simulink model "Test_SG_circuit_exc_turb"  (R2020b)
settings: Solver=ode1  StartTime=0.0  StopTime=15  FixedStep=10e-6  RelTol=1e-3
values from neighbouring files (symbols this model uses):
  L1d_pu = Lb/Lbase    [SG_param.m]    (also in SG_param_tool.m; SG_param_tool_POD.m = (Xd_subtr-Xl)*(Lmd_pu*Lfd_pu)/(Lmd_pu*Lfd_pu-(Lfd_pu+Lmd_pu))
  L1q_pu = La/Lbase    [SG_param.m]    (also in SG_param_tool.m; SG_param_tool_POD.m = (Lmq_pu*(Xq_tr-Xl))/(Lmq_pu-Xq_tr+Xl))
  L2q_pu = Lb/Lbase    [SG_param.m]    (also in SG_param_tool.m; SG_param_tool_POD.m = (Xq_subtr-Xl)*(Lmq_pu*L1q_pu)/(Lmq_pu*L1q_pu-(L1q_pu+Lmq_pu))
  Lfd_pu = La/Lbase    [SG_param.m]    (also in SG_param_tool.m; SG_param_tool_POD.m = (Lmd_pu*(Xd_tr-Xl))/(Lmd_pu-Xd_tr+Xl))
  Ll_pu = Xl    (= 0.2)    [SG_param.m]    (also in SG_param_tool.m; SG_param_tool_POD.m = Xl)
  Lmd_pu = Xd - Xl    (= 1.6)    [SG_param.m]    (also in SG_param_tool.m; SG_param_tool_POD.m = Xd - Xl)
  Lmq_pu = Xq - Xl    (= 1.5)    [SG_param.m]    (also in SG_param_tool.m; SG_param_tool_POD.m = Xq - Xl)
  Pm = Psg0+(Iq.^2+Id.^2)*Rs_pu    [Init_values_Simulink.m]    (also in Init_values_Simulink_trafo.m)
  R1d_pu = rb/Zb    [SG_param.m]    (also in SG_param_tool.m; SG_param_tool_POD.m = 1/(Tdo_subtr*wb)*(L1d_pu+Lmd_pu*Lfd_pu/(Lmd_pu+Lfd_pu)))
  R1q_pu = ra/Zb    [SG_param.m]    (also in SG_param_tool.m; SG_param_tool_POD.m = (Lmq_pu+L1q_pu)/(Tqo_tr*wb))
  R2q_pu = rb/Zb    [SG_param.m]    (also in SG_param_tool.m; SG_param_tool_POD.m = 1/(Tqo_subtr*wb)*(L2q_pu+Lmq_pu*L1q_pu/(Lmq_pu+L1q_pu)))
  Rf_pu = ra/Zb    [SG_param.m]    (also in SG_param_tool.m; SG_param_tool_POD.m = (Lmd_pu+Lfd_pu)/(Tdo_tr*wb))
  Rs_pu = 0.0025    [SG_param.m]    (also in SG_param_tool.m; SG_param_tool_POD.m)
  Rsnb = 300    [SG_param.m]    (also in SG_param_tool.m; SG_param_tool_POD.m; SS_model_grid.m = Vn^2/(data.SG(ii,2)*1e6*0.01)*Ssnb(ii))
  Vb = 22e3    (= 22000)    [SG_param.m]    (also in sg_slack_POD.m = Vb_kV*1e3)
  Vf = Efd    [Init_values_Simulink.m]    (also in Init_values_Simulink_trafo.m)
  Vref = Efd/Exc.KA+V    [Init_values_Simulink.m]    (also in Init_values_Simulink_trafo.m = Vf/Exc.KA+V; Initial_values_for_linear_model.m = Efd/Exc.KA+abs(Vin))
  wn = 2*pi*fn    (= 314.159265359)    [SG_param.m]
undefined symbols (not defined in the file or in its folder): Exc, Lg, Rg, tstep
libraries: powerlib x41, simulink_extras x9, powerlib_meascontrol x2
(part 1 of 2)
settings Model: Creator=Usuario  LastModifiedBy=Collados

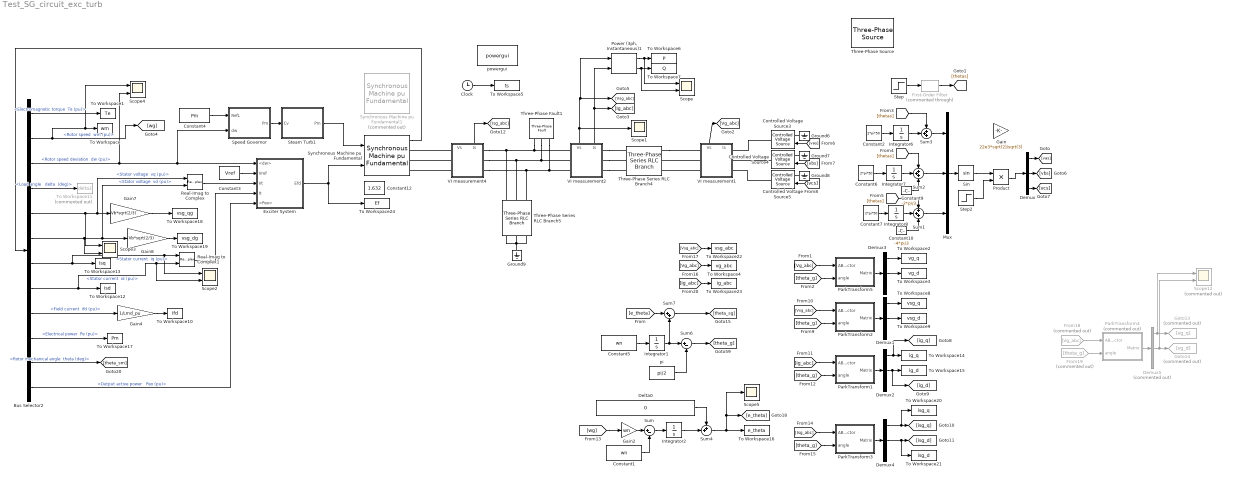
== system Test_SG_circuit_exc_turb ==
  Bus Selector2 : BusSelector  OutputSignals="Mechanical.Electromagnetic torque  Te (pu),Mechanical.Rotor speed  wm (pu),Mechanical.Rotor speed deviation  dw (pu),Load angle   delta  (deg),dq0 components.Stator voltage  vq (pu),dq0 components.Stator voltage  vd (pu),dq0 components.Stator current  iq (pu),dq0 components.Stator current  id (pu),dq0 components.Field current  ifd (pu),Mechanical.Electrical power  Pe (pu),Mechanical.Rotor mechanical angle  theta (deg),Output active power   Peo (pu)"
  Clock : Clock
  Constant1 : Constant  Value=wn
  Constant10 : Constant  Value=-4*pi/3
  Constant12 : Constant  Value=1.632
  Constant2 : Constant  Value=2*pi*50
  Constant3 : Constant  Value=Vref
  Constant4 : Constant  Value=Pm
  Constant5 : Constant  Value=wn
  Constant6 : Constant  Value=2*pi*50
  Constant7 : Constant  Value=2*pi*50
  Constant9 : Constant  Value=-2*pi/3
  Controlled Voltage Source3 : powerlib/Electrical Sources/Controlled Voltage Source  Initialize=on  Source_Type=AC  Amplitude=0  Phase=0  Frequency=0  Measurements=None
  Controlled Voltage Source4 : powerlib/Electrical Sources/Controlled Voltage Source  Initialize=on  Source_Type=AC  Amplitude=0  Phase=0  Frequency=0  Measurements=None
  Controlled Voltage Source5 : powerlib/Electrical Sources/Controlled Voltage Source  Initialize=on  Source_Type=AC  Amplitude=0  Phase=0  Frequency=0  Measurements=None
  Delta0 : Constant  Value=0
  Demux{,1..4} (5 alike) : Demux  Outputs=3
  Demux5 : Demux  Commented=on  Outputs=3
  Exciter System : Subsystem
  First-Order Filter : powerlib_meascontrol/Filters/First-Order Filter  Commented=through  FilterType=Lowpass  Tc=41.4e-3  Ts=0  Initialize=off  Vac_Init=[0, 0, 60]  Vdc_Init=0  PlotResponse=off  FreqRange="[0,  200,  1]"
  From18 : From  Commented=on  GotoTag=Vg_abc
  From19 : From  Commented=on  GotoTag=theta_g
  Gain : Gain  Gain=22e3*sqrt(2)/sqrt(3)
  Gain2 : Gain  Gain=wn
  Gain4 : Gain  Gain=1/Lmd_pu
  Gain7 : Gain  Gain=Vb*sqrt(2/3)
  Gain8 : Gain  Gain=Vb*sqrt(2/3)
  Goto13 : Goto  Commented=on  GotoTag=vg_q
  Goto14 : Goto  Commented=on  GotoTag=vg_d
  Ground{6..9} (4 alike) : powerlib/Elements/Ground  LConnTagsString=a
  Integrator{1..2,6..8} (5 alike) : Integrator
  Mux : Mux  Inputs=3
  ParkTransform1 : Subsystem  mask(Gerard){}
      mask help:
      | This block applies the park transfomation from a desired vector.
      | The input Xabc refers to the vector in the ABC frame, and the second input is the angle used in the transformation.
      | The output is the vector in the qd0 frame.
      mask Display:
      | port_label('output',1,'Xqd0')
      | port_label('input',1,'Xabc')
      | port_label('input',2,'angle')
  ParkTransform2 : Subsystem  mask(Gerard){}
      mask help:
      | This block applies the park transfomation from a desired vector.
      | The input Xabc refers to the vector in the ABC frame, and the second input is the angle used in the transformation.
      | The output is the vector in the qd0 frame.
      mask Display:
      | port_label('output',1,'Xqd0')
      | port_label('input',1,'Xabc')
      | port_label('input',2,'angle')
  ParkTransform3 : Subsystem  mask(Gerard){}
      mask help:
      | This block applies the park transfomation from a desired vector.
      | The input Xabc refers to the vector in the ABC frame, and the second input is the angle used in the transformation.
      | The output is the vector in the qd0 frame.
      mask Display:
      | port_label('output',1,'Xqd0')
      | port_label('input',1,'Xabc')
      | port_label('input',2,'angle')
  ParkTransform4 : Subsystem  Commented=on  mask(Gerard){}
      mask help:
      | This block applies the park transfomation from a desired vector.
      | The input Xabc refers to the vector in the ABC frame, and the second input is the angle used in the transformation.
      | The output is the vector in the qd0 frame.
      mask Display:
      | port_label('output',1,'Xqd0')
      | port_label('input',1,'Xabc')
      | port_label('input',2,'angle')
  ParkTransform5 : Subsystem  mask(Gerard){}
      mask help:
      | This block applies the park transfomation from a desired vector.
      | The input Xabc refers to the vector in the ABC frame, and the second input is the angle used in the transformation.
      | The output is the vector in the qd0 frame.
      mask Display:
      | port_label('output',1,'Xqd0')
      | port_label('input',1,'Xabc')
      | port_label('input',2,'angle')
  "Power (3ph, Instantaneous)1" : powerlib_meascontrol/Measurements/Power (3ph, Instantaneous)
  Product : Product
  Real-Imag to Complex : RealImagToComplex
  Real-Imag to Complex1 : RealImagToComplex
  Scope{,2..4} (4 alike) : Scope  NumInputPorts=2
  Scope1 : Scope
  Scope12 : Scope  Commented=on  NumInputPorts=2
  Scope5 : Scope
  Sin : Trigonometry
  Speed Governor : Subsystem  mask{R=0.05, T1=0.5, T2=3, T3=10, Dt=0, Vmin=0, Vmax=10, P0=Pm}
      mask prompts: R "Controller droop (R)"; T1 "Governor time constant (T1)(sec)"; T2 "Turbine derivative time constant (T2)(sec)"; T3 "Turbine delay time constant (T3)(sec)"; Dt "Frictional losses factor (Dt)"; Vmin "Minimum gate limit (Vmin)(p.u)"; Vmax "Maximum gate limit (Vmax)(p.u)"; P0 "Initial power (p.u)"
      mask Display:
      | disp('TGOV')
      | 
      | port_label('input',1,'Pref')
      | port_label('input',2,'dw')
      | 
      | port_label('output',1,'Cv')
  Steam Turb1 : Subsystem  mask{K1=0.22, K3=0, K5=0.14, K7=0.14, K2=0, K4=0.22, K6=0.14, K8=0.14, T4=0.25, T5=7.5, T6=7.5, T7=0.4, P0=Pm}
      mask prompts: K1 "K1 fraction (HP Turbine)(pu)"; K3 "K3 fraction (HP Turbine)(pu)"; K5 "K5 fraction (HP Turbine)(pu)"; K7 "K7 fraction (HP Turbine)(pu)"; K2 "K2 fraction (LP Turbine)(pu)"; K4 "K4 fraction (LP Turbine)(pu)"; K6 "K6 fraction (LP Turbine)(pu)"; K8 "K8 fraction (LP Turbine)(pu)"; T4 "Steam chest time constant (T4)(sec)"; T5 "Reheater time constant (T5)(sec)"; T6 "Reheater/cross-over time constant (T6)(sec)"; T7 "Cross-over time constant (T7)(sec)"; P0 "Initial power (p.u)"
      mask Display:
      | disp('TTurb')
      | 
      | port_label('input',1,'Cv')
      | 
      | port_label('output',1,'Pm')
  Step : Step  Time=tstep+100  After=10*pi/180  SampleTime=0
  Step2 : Step  Time=tstep  Before=22e3*sqrt(2)/sqrt(3)  After=22e3*sqrt(2)/sqrt(3)*1.005  SampleTime=0
  Sum : Sum  Inputs=|+-
  Sum1 : Sum  Inputs=+++
  Sum2 : Sum  Inputs=+++
  Sum3 : Sum  Inputs=+++
  Sum4 : Sum  Inputs=++|
  Sum6 : Sum  Inputs=|+-
  Sum7 : Sum  Inputs=|++
  Synchronous Machine pu Fundamental : powerlib/Machines/Synchronous Machine pu Fundamental  PresetModel=No  MechanicalLoad=Mechanical power Pm  ShowDetailedParameters=on  RotorType=Round  Units=per unit fundamental parameters  MeasurementBus=off  NominalParameters="[100e6  22e3   50]"  Stator="[Rs_pu  Ll_pu  Lmd_pu  Lmq_pu ]"  Field="[ Rf_pu  Lfd_pu]"  Dampers2=[R1d_pu, L1d_pu, R1q_pu, L1q_pu, R2q_pu, L2q_pu ]  Dampers1="[ 1.17E-02  0.182  1.97E-02  0.384 ]"  Mechanical=[ 5 0 1]  PolePairs=20  InitialConditions=init_values_SG  SetSaturation=off  Saturation=[0.6404,0.7127,0.8441,0.9214,0.9956,1.082,1.19,1.316,1.457;0.7,0.7698,0.8872,0.9466,0.9969,1.046,1.1,1.151,1.201]  LoadFlowParameters=[1,0,0,0,0]  TsPowergui=0  TsBlock=-1  IterativeModel=Trapezoidal non iterative  IterativeDiscreteModel=Trapezoidal non iterative  BusType=PQ  Pref=50e6  Qref=20e6  Qmin=-inf  Qmax=inf  PLF=0  QLF=0
      settings: SourceProductBaseCode=PS
  Synchronous Machine pu Fundamental1 : powerlib/Machines/Synchronous Machine pu Fundamental  Commented=on  PresetModel=No  MechanicalLoad=Mechanical power Pm  ShowDetailedParameters=on  RotorType=Round  Units=per unit fundamental parameters  MeasurementBus=off  NominalParameters="[100e6  22e3   50]"  Stator="[ 0.0025  0.14  1.66  0.91 ]"  Field="[ 0.00043  0.2004]"  Dampers2=[0.0051, 0.0437, 0.00842, 0.106, 8.1942e-3, 9.4199e-2 ]  Dampers1="[ 1.17E-02  0.182  1.97E-02  0.384 ]"  Mechanical=[ 5 0 2]  PolePairs=20  InitialConditions=[0 -78.0791 0.205424 0.205424 0.205424 -13.3134 -133.313 106.687 1.14256]  SetSaturation=off  Saturation=[0.6404,0.7127,0.8441,0.9214,0.9956,1.082,1.19,1.316,1.457;0.7,0.7698,0.8872,0.9466,0.9969,1.046,1.1,1.151,1.201]  LoadFlowParameters=[1,0,0,0,0]  TsPowergui=0  TsBlock=-1  IterativeModel=Trapezoidal non iterative  IterativeDiscreteModel=Trapezoidal non iterative  BusType=PQ  Pref=20e6  Qref=5e6  Qmin=-inf  Qmax=inf  PLF=0  QLF=0
      settings: SourceProductBaseCode=PS
  Three-Phase Series RLC Branch4 : powerlib/Elements/Three-Phase Series RLC Branch  LConnTagsString=A|B|C  RConnTagsString=A|B|C  BranchType=RL  Resistance=Rg  Inductance=Lg  Capacitance=1e-6  Measurements=None
  Three-Phase Series RLC Branch5 : powerlib/Elements/Three-Phase Series RLC Branch  LConnTagsString=A|B|C  RConnTagsString=A|B|C  BranchType=R  Resistance=Rsnb  Inductance=1e-3  Capacitance=1e-6  Measurements=None
  Three-Phase Fault1 : powerlib/Elements/Three-Phase Fault  InitialStates=0  FaultA=on  FaultB=off  FaultC=off  GroundFault=on  SwitchTimes=[101 101.2]  External=off  SwitchStatus=NaN  FaultResistance=50  GroundResistance=0.0000001  SnubberResistance=1e6  SnubberCapacitance=inf  Measurements=None
  Three-Phase Source : powerlib/Electrical Sources/Three-Phase Source  InternalConnection=Yg  VoltagePhases=off  Voltage=(22000)*1  PhaseAngle=0  Voltage_phases=[25e3 25e3 25e3]/sqrt(3)  PhaseAngles_phases=[0 -120 +120]  Frequency=50  NonIdealSource=off  SpecifyImpedance=off  Resistance=0.8929  Inductance=16.58e-3  ShortCircuitLevel=100e6  BaseVoltage=22e3  XRratio=7  BusType=swing  Pref=10e3  Qref=0  Prefabc=[10e3, 10e3, 10e3]  Qrefabc=[0, 0, 0]  Qmin=-inf  Qmax=inf
  To Workspace : ToWorkspace  VariableName=wm  SampleTime=-1
      settings: Decimation=20  Save2DSignal=2-D array (concatenate along first dimension)
  To Workspace1 : ToWorkspace  VariableName=Te  SampleTime=-1
      settings: Decimation=20  Save2DSignal=2-D array (concatenate along first dimension)
  To Workspace10 : ToWorkspace  VariableName=ifd  SampleTime=-1
      settings: Decimation=20  Save2DSignal=2-D array (concatenate along first dimension)
  To Workspace11 : ToWorkspace  Commented=on  VariableName=delta2  SampleTime=-1
      settings: Decimation=20  Save2DSignal=2-D array (concatenate along first dimension)
  To Workspace12 : ToWorkspace  VariableName=isd  SampleTime=-1
      settings: Decimation=20  Save2DSignal=2-D array (concatenate along first dimension)
  To Workspace13 : ToWorkspace  VariableName=isq  SampleTime=-1
      settings: Decimation=20  Save2DSignal=2-D array (concatenate along first dimension)
  To Workspace14 : ToWorkspace  VariableName=ig_q  SampleTime=-1
      settings: Decimation=20  Save2DSignal=2-D array (concatenate along first dimension)
  To Workspace15 : ToWorkspace  VariableName=ig_d  SampleTime=-1
      settings: Decimation=20  Save2DSignal=2-D array (concatenate along first dimension)
  To Workspace16 : ToWorkspace  VariableName=e_theta  SampleTime=-1
      settings: Decimation=20  Save2DSignal=2-D array (concatenate along first dimension)
  To Workspace17 : ToWorkspace  VariableName=Pm  SampleTime=-1
      settings: Decimation=20  Save2DSignal=2-D array (concatenate along first dimension)
  To Workspace18 : ToWorkspace  VariableName=vsg_qg  SampleTime=-1
      settings: Decimation=20  Save2DSignal=2-D array (concatenate along first dimension)
  To Workspace19 : ToWorkspace  VariableName=vsg_dg  SampleTime=-1
      settings: Decimation=20  Save2DSignal=2-D array (concatenate along first dimension)
  To Workspace2 : ToWorkspace  VariableName=vg_q  SampleTime=-1
      settings: Decimation=20  Save2DSignal=2-D array (concatenate along first dimension)
  To Workspace20 : ToWorkspace  VariableName=isg_q  SampleTime=-1
      settings: Decimation=20  Save2DSignal=2-D array (concatenate along first dimension)
  To Workspace21 : ToWorkspace  VariableName=isg_d  SampleTime=-1
      settings: Decimation=20  Save2DSignal=2-D array (concatenate along first dimension)
  To Workspace22 : ToWorkspace  VariableName=vsg_abc  SampleTime=-1
      settings: Decimation=20  Save2DSignal=2-D array (concatenate along first dimension)
  To Workspace23 : ToWorkspace  VariableName=ig_abc  SampleTime=-1
      settings: Decimation=20  Save2DSignal=2-D array (concatenate along first dimension)
  To Workspace24 : ToWorkspace  VariableName=Ef  SampleTime=-1
      settings: Decimation=20  Save2DSignal=2-D array (concatenate along first dimension)
  To Workspace3 : ToWorkspace  VariableName=vg_d  SampleTime=-1
      settings: Decimation=20  Save2DSignal=2-D array (concatenate along first dimension)
  To Workspace4 : ToWorkspace  VariableName=vg_abc  SampleTime=-1
      settings: Decimation=20  Save2DSignal=2-D array (concatenate along first dimension)
  To Workspace5 : ToWorkspace  VariableName=ts  SampleTime=-1
      settings: Decimation=20  Save2DSignal=2-D array (concatenate along first dimension)
  To Workspace6 : ToWorkspace  VariableName=P  SampleTime=-1
      settings: Decimation=20  Save2DSignal=2-D array (concatenate along first dimension)
  To Workspace7 : ToWorkspace  VariableName=Q  SampleTime=-1
      settings: Decimation=20  Save2DSignal=2-D array (concatenate along first dimension)
  To Workspace8 : ToWorkspace  VariableName=vsg_q  SampleTime=-1
      settings: Decimation=20  Save2DSignal=2-D array (concatenate along first dimension)
  To Workspace9 : ToWorkspace  VariableName=vsg_d  SampleTime=-1
      settings: Decimation=20  Save2DSignal=2-D array (concatenate along first dimension)
  VI measurement1 : Subsystem
      settings: PortSchema="{\"entries\":[{\"content\":{\"sides\":[{\"content\":{\"connectorIds\":[\"LConn1\",\"LConn2\",\"LConn3\"]},\"type\":\"ConnectorPlacement.EquallySpacedRectSide\",\"uuid\":\"d0d5b0b8-afec-4f90-9eba-536a06b10059\"},{\"content\":{\"connectorIds\":[\"RConn1\",\"RConn2\",\"RConn3\"],\"side\":\"RIGHT\"},\"type\":\"ConnectorPlacement.EquallySpacedRectSide\",\"uuid\":\"adc1b68d-6172-4507-b54b-9373921355a1\"},{\"content\":{\"connectorIds\":[\"Out1\",\"Out2\"],\"side\":\"TOP\"},\"type\":\"ConnectorPlacement.EquallySpacedRectSide\",\"uuid\":\"8c5adf07-e95b-4907-94c3-1b2a47d47f40\"}]},\"type\":\"ConnectorPlacement.EquallySpacedConnector\",\"uuid\":\"87d0b20f-8f85-4790-a611-3415e642a83a\"}],\"packageUris\":[\"http://schema.mathworks.com/mf0/Connector/R2020b\"],\"version\":\"1.0\"}"
  VI measurement2 : Subsystem
      settings: PortSchema="{\"entries\":[{\"content\":{\"sides\":[{\"content\":{\"connectorIds\":[\"LConn1\",\"LConn2\",\"LConn3\"]},\"type\":\"ConnectorPlacement.EquallySpacedRectSide\",\"uuid\":\"d0d5b0b8-afec-4f90-9eba-536a06b10059\"},{\"content\":{\"connectorIds\":[\"RConn1\",\"RConn2\",\"RConn3\"],\"side\":\"RIGHT\"},\"type\":\"ConnectorPlacement.EquallySpacedRectSide\",\"uuid\":\"adc1b68d-6172-4507-b54b-9373921355a1\"},{\"content\":{\"connectorIds\":[\"Out1\",\"Out2\"],\"side\":\"TOP\"},\"type\":\"ConnectorPlacement.EquallySpacedRectSide\",\"uuid\":\"8c5adf07-e95b-4907-94c3-1b2a47d47f40\"}]},\"type\":\"ConnectorPlacement.EquallySpacedConnector\",\"uuid\":\"87d0b20f-8f85-4790-a611-3415e642a83a\"}],\"packageUris\":[\"http://schema.mathworks.com/mf0/Connector/R2020b\"],\"version\":\"1.0\"}"
  VI measurement4 : Subsystem
      settings: PortSchema="{\"entries\":[{\"content\":{\"sides\":[{\"content\":{\"connectorIds\":[\"LConn1\",\"LConn2\",\"LConn3\"]},\"type\":\"ConnectorPlacement.EquallySpacedRectSide\",\"uuid\":\"d0d5b0b8-afec-4f90-9eba-536a06b10059\"},{\"content\":{\"connectorIds\":[\"RConn1\",\"RConn2\",\"RConn3\"],\"side\":\"RIGHT\"},\"type\":\"ConnectorPlacement.EquallySpacedRectSide\",\"uuid\":\"adc1b68d-6172-4507-b54b-9373921355a1\"},{\"content\":{\"connectorIds\":[\"Out1\",\"Out2\"],\"side\":\"TOP\"},\"type\":\"ConnectorPlacement.EquallySpacedRectSide\",\"uuid\":\"8c5adf07-e95b-4907-94c3-1b2a47d47f40\"}]},\"type\":\"ConnectorPlacement.EquallySpacedConnector\",\"uuid\":\"87d0b20f-8f85-4790-a611-3415e642a83a\"}],\"packageUris\":[\"http://schema.mathworks.com/mf0/Connector/R2020b\"],\"version\":\"1.0\"}"
  pi : Constant  Value=pi/2
  powergui : powerlib/powergui  Priority=1  SimulationMode=Discrete  SampleTime=10e-6  frequency=60  Iterations=50  frequencyindice=0  Pbase=100e6  ErrMax=0.0001  UnitsV=kV  UnitsW=MW  buscounter=0  FunctionMessages=off  echomessages=off  EnableUseOfTLC=off  CurrentSourceSwitches=off  DisableSnubberDevices=off  DisableRonSwitches=off  DisableVfSwitches=off  DisplayEquations=off  AutomaticDiscreteSolvers=off  SolverType=Tustin/Backward Euler (TBE)  Interpol=off  ExternalGateDelay=off  methode=off  Ts=100  x0status=blocks  SPID=on  SwTol=0  HookPort=off  NonlinearTolerance=1e-4  nMaxIteration=100  ContinueOnMaxIteration=off  RestoreLinks=warning  ResistiveCurrentMeasurement=off  Frange=[0:2:500]  Ylog=off  Xlog=on  ShowGrid=off  save=off  variable=ZData  structure=0  ZoomFFT=off  StartTime=0.0  cycles=1  DisplayStyle=1  fundamental=60  FreqAxis=off  MaxFrequency=1000  frequencyindicesteady=1  RmsSteady=1  display=off
  wires:
  Constant6/1 -> Integrator7/1
  Demux/3 -> [vcs]
  Demux/1 -> [vas]
  Constant7/1 -> Integrator8/1
  Demux/2 -> [vbs]
  Sum2/1 -> Mux/2
  Sin/1 -> Product/1
  Product/1 -> Demux/1
  Sum1/1 -> Mux/3
  Mux/1 -> Sin/1
  Constant2/1 -> Integrator6/1
  Constant9/1 -> Sum2/3
  Integrator7/1 -> Sum2/2
  Integrator6/1 -> Sum3/2
  [thetas] -> Sum3/1
  [thetas] -> Sum2/1
  Integrator8/1 -> Sum1/2
  Constant10/1 -> Sum1/3
  [thetas] -> Sum1/1
  Sum3/1 -> Mux/1
  Step/1 -> First-Order Filter/1
  First-Order Filter/1 -> [thetas]
  Clock/1 -> To Workspace5/1
  Steam Turb1/1(Pm) -> Synchronous Machine pu Fundamental/1
  [vas] -> Controlled Voltage Source3/1
  [vcs] -> Controlled Voltage Source5/1
  [vbs] -> Controlled Voltage Source4/1
  VI measurement2/2(Is) -> "Power (3ph, Instantaneous)1"/2, [Ig_abc]
  Constant5/1 -> Integrator1/1
  ParkTransform2/1(Matrix) -> Demux1/1
  Integrator1/1 -> Sum6/1, Sum7/2
  [theta_g] -> ParkTransform2/2(angle)
  [Vsg_abc] -> ParkTransform2/1(ABC vector)
  Demux1/2 -> To Workspace9/1
  Demux1/1 -> To Workspace8/1
  Demux2/1 -> [ig_q], To Workspace14/1
  Demux2/2 -> [ig_d], To Workspace15/1
  [Ig_abc] -> ParkTransform1/1(ABC vector)
  [theta_g] -> ParkTransform1/2(angle)
  ParkTransform1/1(Matrix) -> Demux2/1
  VI measurement2/1(Vs) -> Scope1/1, "Power (3ph, Instantaneous)1"/1, [Vsg_abc]
  "Power (3ph, Instantaneous)1"/1 -> Scope/1, To Workspace6/1
  "Power (3ph, Instantaneous)1"/2 -> Scope/2, To Workspace7/1
  [wg] -> Gain2/1
  Sum/1 -> Integrator2/1
  Integrator2/1 -> Sum4/2
  Gain2/1 -> Sum/1
  Sum4/1 -> Scope5/1, [e_theta], To Workspace16/1
  ParkTransform3/1(Matrix) -> Demux4/1
  [theta_g] -> ParkTransform3/2(angle)
  [Isg_abc] -> ParkTransform3/1(ABC vector)
  Demux4/2 -> To Workspace21/1, [isg_d]
  Demux4/1 -> To Workspace20/1, [isg_q]
  VI measurement4/2(Is) -> [Isg_abc]
  From18/1 -> ParkTransform4/1(ABC vector)
  From19/1 -> ParkTransform4/2(angle)
  ParkTransform4/1(Matrix) -> Demux5/1
  Demux5/1 -> Scope12/1, Goto13/1
  Demux5/2 -> Scope12/2, Goto14/1
  pi/1 -> Sum6/2
  Sum6/1 -> [theta_g]
  Sum7/1 -> [theta_sg]
  Step2/1 -> Product/2
  Delta0/1 -> Sum4/1
  Constant1/1 -> Sum/2
  [e_theta] -> Sum7/1
  VI measurement1/1(Vs) -> [Vg_abc]
  Demux3/1 -> To Workspace2/1
  Demux3/2 -> To Workspace3/1
  [Vg_abc] -> ParkTransform5/1(ABC vector)
  [theta_g] -> ParkTransform5/2(angle)
  ParkTransform5/1(Matrix) -> Demux3/1
  [Vg_abc] -> To Workspace4/1
  [Vsg_abc] -> To Workspace22/1
  [Ig_abc] -> To Workspace23/1
  Bus Selector2/10 -> To Workspace17/1  "<Electrical power  Pe (pu)>"
  Real-Imag to Complex1/1 -> Exciter System/4(It)
  Gain7/1 -> To Workspace18/1
  Bus Selector2/9 -> Gain4/1  "<Field current  ifd (pu)>"
  Constant3/1 -> Exciter System/2(Vref)
  Bus Selector2/6 -> Scope3/2, Real-Imag to Complex/2, Gain8/1  "<Stator voltage  vd (pu)>"
  Bus Selector2/1 -> To Workspace1/1  "<Electromagnetic torque  Te (pu)>"
  Bus Selector2/5 -> Scope3/1, Real-Imag to Complex/1, Gain7/1  "<Stator voltage  vq (pu)>"
  Bus Selector2/7 -> Scope2/1, Real-Imag to Complex1/1, To Workspace13/1  "<Stator current  iq (pu)>"
  Bus Selector2/4 -> To Workspace11/1  "<Load angle   delta  (deg)>"
  Synchronous Machine pu Fundamental/1 -> Bus Selector2/1
  Bus Selector2/2 -> Scope4/1, To Workspace/1, [wg]  "<Rotor speed  wm (pu)>"
  Bus Selector2/11 -> [theta_sm]  "<Rotor mechanical angle  theta (deg)>"
  Real-Imag to Complex/1 -> Exciter System/3(Vt)
  Gain8/1 -> To Workspace19/1
  Gain4/1 -> To Workspace10/1
  Bus Selector2/8 -> Scope2/2, Real-Imag to Complex1/2, To Workspace12/1  "<Stator current  id (pu)>"
  Bus Selector2/12 -> Exciter System/5(<Peo>)  "<Output active power   Peo (pu)>"
  Exciter System/1(Efd) -> Synchronous Machine pu Fundamental/2, To Workspace24/1
  Constant4/1 -> Speed Governor/1(RefL)
  Bus Selector2/3 -> Scope4/2, Speed Governor/2(dw), Exciter System/1(<dw>)  "<Rotor speed deviation  dw (pu)>"
  Speed Governor/1(Pm) -> Steam Turb1/1(Cv)
  connections:
  Three-Phase Fault1/LConn1 -- VI measurement2/LConn1 -- Three-Phase Series RLC Branch5/LConn1 -- VI measurement4/RConn1
  Three-Phase Series RLC Branch5/RConn1 -- Ground9/LConn1 -- Three-Phase Series RLC Branch5/RConn2 -- Three-Phase Series RLC Branch5/RConn3
  Ground6/LConn1 -- Controlled Voltage Source3/LConn1
  VI measurement2/RConn2 -- Three-Phase Series RLC Branch4/LConn2
  Ground7/LConn1 -- Controlled Voltage Source4/LConn1
  Ground8/LConn1 -- Controlled Voltage Source5/LConn1
  VI measurement2/RConn3 -- Three-Phase Series RLC Branch4/LConn3
  VI measurement2/RConn1 -- Three-Phase Series RLC Branch4/LConn1
  VI measurement4/LConn1 -- Synchronous Machine pu Fundamental/RConn1
  VI measurement4/LConn2 -- Synchronous Machine pu Fundamental/RConn2
  VI measurement4/LConn3 -- Synchronous Machine pu Fundamental/RConn3
  VI measurement4/RConn2 -- VI measurement2/LConn2 -- Three-Phase Fault1/LConn2 -- Three-Phase Series RLC Branch5/LConn2
  VI measurement4/RConn3 -- VI measurement2/LConn3 -- Three-Phase Fault1/LConn3 -- Three-Phase Series RLC Branch5/LConn3
  Three-Phase Series RLC Branch4/RConn1 -- VI measurement1/LConn1
  Controlled Voltage Source3/RConn1 -- VI measurement1/RConn1
  Controlled Voltage Source4/RConn1 -- VI measurement1/RConn2
  Controlled Voltage Source5/RConn1 -- VI measurement1/RConn3
  VI measurement1/LConn2 -- Three-Phase Series RLC Branch4/RConn2
  VI measurement1/LConn3 -- Three-Phase Series RLC Branch4/RConn3

== system Test_SG_circuit_exc_turb/Exciter System ==
  <dw> : Inport
  Vref : Inport  Port=2
  Vt : Inport  Port=3
  It : Inport  Port=4
  <Peo> : Inport  Port=5
  PSS1 : Subsystem  mask{Ks1=20, Ks2=0.1564, Ks3=1, Tw1=2, Tw2=2, Tw3=2, Tw4=0, T1=0.25, T2=0.2, T3=0.15, T4=0.1, T6=0, T7=2, T8=0.5, T9=0.1, Vstmin=-0.10, Vstmax=0.10, N=1, M=1, IC1=1, IC2=3}
      mask prompts: Ks1 "PSS gain (Ks1)"; Ks2 "2nd signal transducer factor(Ks2)"; Ks3 "washouts coupling factor (Ks3)"; Tw1 "1st washout 1th time constant (Tw1)(sec)"; Tw2 "1st washout 2nd time constant (Tw2)(sec)"; Tw3 "2nd washout 1st time constant (Tw3)(sec)"; Tw4 "2nd washout 2nd time constant (Tw4)(sec)"; T1 "1st lead-lag derivative time constant (T1)(sec)"; T2 "1st lead-lag delay time constant(T2)(sec)"; T3 "2nd lead-lag derivative time constant(T3)(sec)"; T4 "2nd lead-lag delay time constant(T4)(sec)"; T6 "1st signal transducer time constant(T6)(sec)"; T7 "2nd signal transducer time constant(T7)(sec)"; T8 "ramp tracking filter deriv. time constant(T8)(sec)"; T9 "ramp tracking filter delay time constant(T9)(sec)"; Vstmin "controller minimum output(Vstmin)"; Vstmax "controller maximum output(Vstmax)"; N "ramp tracking filter (N)"; M "ramp tracking filter (M)"; IC1 "1st input selector (IC1)"; IC2 "2nd input selector (IC2)"
      mask Display:
      | disp('PSS2A')
      | 
      | port_label('input',1,'dw')
      | port_label('input',2,'Pg')
      | %port_label('input',3,'Vs')
      | 
      | port_label('output',1,'Vs')
  PSS1 backup : Subsystem  Commented=on  mask{Ks1=10, Ks2=0.1564, Ks3=1, Tw1=2, Tw2=2, Tw3=2, Tw4=0, T1=0.25, T2=0.03, T3=0.15, T4=0.015, T6=0, T7=2, T8=0.5, T9=0.1, Vstmin=-0.1, Vstmax=0.1, N=0, M=0, IC1=1, IC2=3}
      mask prompts: Ks1 "PSS gain (Ks1)"; Ks2 "2nd signal transducer factor(Ks2)"; Ks3 "washouts coupling factor (Ks3)"; Tw1 "1st washout 1th time constant (Tw1)(sec)"; Tw2 "1st washout 2nd time constant (Tw2)(sec)"; Tw3 "2nd washout 1st time constant (Tw3)(sec)"; Tw4 "2nd washout 2nd time constant (Tw4)(sec)"; T1 "1st lead-lag derivative time constant (T1)(sec)"; T2 "1st lead-lag delay time constant(T2)(sec)"; T3 "2nd lead-lag derivative time constant(T3)(sec)"; T4 "2nd lead-lag delay time constant(T4)(sec)"; T6 "1st signal transducer time constant(T6)(sec)"; T7 "2nd signal transducer time constant(T7)(sec)"; T8 "ramp tracking filter deriv. time constant(T8)(sec)"; T9 "ramp tracking filter delay time constant(T9)(sec)"; Vstmin "controller minimum output(Vstmin)"; Vstmax "controller maximum output(Vstmax)"; N "ramp tracking filter (N)"; M "ramp tracking filter (M)"; IC1 "1st input selector (IC1)"; IC2 "2nd input selector (IC2)"
      mask Display:
      | disp('PSS2A')
      | 
      | port_label('input',1,'dw')
      | port_label('input',2,'Pg')
      | %port_label('input',3,'Vs')
      | 
      | port_label('output',1,'Vs')
  SEXS1 : Subsystem  mask{K=Exc.KA, Ta=Exc.TC, Tb=Exc.TB, Te=Exc.TA, Emin=Exc.VRmin, Emax=Exc.VRmax, Vf0=Vf}
      mask prompts: K "Controller gain (K)"; Ta "Filter derivative time constant (Ta)(sec)"; Tb "Filter delay time (Tb)(sec)"; Te "Exciter time constant (Te)(sec)"; Emin "Controller minimum output (Emin)"; Emax "Controller maximum output (Emax)"; Vf0 "Initial value of field voltage"
      mask Display:
      | disp('AVR')
      | 
      | port_label('input',1,'Vref')
      | port_label('input',2,'Vc')
      | port_label('input',3,'Vs')
      | 
      | port_label('output',1,'Efd')
  TR and LC_test : Subsystem  mask{Tr=10e-3, Rc=0, Xc=0}
      mask prompts: Tr "Transducter filter time constant (Tr)(sec)"; Rc "Resistance to compensate (p.u)"; Xc "Reactance to compensate (p.u)"
      mask Display:
      | %disp('Transducer \n \n')
      | %disp('and \n')
      | %disp('Load compensation')
      | text(15,35, 'Transducer')
      | text(30,24, 'and')
      | text(15,14, 'Load comp')
      | 
      | port_label('input',1,'Vt')
      | port_label('input',2,'It')
      | 
      | port_label('output',1,'Vc')
  To Workspace24 : ToWorkspace  VariableName=Vsg_mag  SampleTime=-1
      settings: Decimation=20  Save2DSignal=2-D array (concatenate along first dimension)
  Efd : Outport
  wires:
  SEXS1/1(Efd) -> Efd/1
  It/1 -> TR and LC_test/2(It)
  PSS1/1(Vothsg) -> ?
  <Peo>/1 -> PSS1/2(Pgen)
  <dw>/1 -> PSS1/1(dw)
  Vt/1 -> TR and LC_test/1(Vt)
  Vref/1 -> SEXS1/1(Vref)
  TR and LC_test/1(Vc) -> To Workspace24/1, SEXS1/2(Vc)

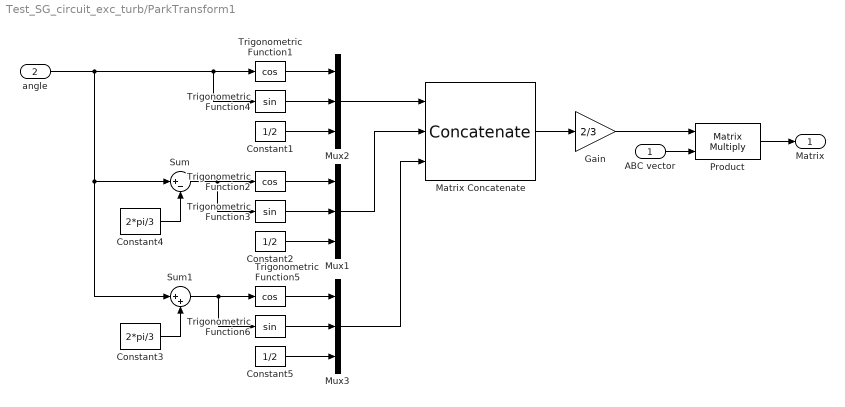
== system Test_SG_circuit_exc_turb/ParkTransform1 ==
  ABC vector : Inport
  angle : Inport  Port=2
  Constant1 : Constant  Value=1/2
  Constant2 : Constant  Value=1/2
  Constant3 : Constant  Value=2*pi/3
  Constant4 : Constant  Value=2*pi/3
  Constant5 : Constant  Value=1/2
  Gain : Gain  Gain=2/3
  Matrix Concatenate : Concatenate  NumInputs=3  Mode=Multidimensional array  ConcatenateDimension=2
  Mux1 : Mux  Inputs=3
  Mux2 : Mux  Inputs=3
  Mux3 : Mux  Inputs=3
  Product : Product  Multiplication=Matrix(*)  RndMeth=Zero
  Sum : Sum  Inputs=|+-
  Sum1 : Sum  Inputs=|++
  Trigonometric Function1 : Trigonometry  Operator=cos
  Trigonometric Function2 : Trigonometry  Operator=cos
  Trigonometric Function3 : Trigonometry
  Trigonometric Function4 : Trigonometry
  Trigonometric Function5 : Trigonometry  Operator=cos
  Trigonometric Function6 : Trigonometry
  Matrix : Outport
  wires:
  Matrix Concatenate/1 -> Gain/1
  ABC vector/1 -> Product/2
  Product/1 -> Matrix/1
  Gain/1 -> Product/1
  Constant4/1 -> Sum/2
  Constant3/1 -> Sum1/2
  angle/1 -> Trigonometric Function4/1, Trigonometric Function1/1, Sum1/1, Sum/1
  Trigonometric Function3/1 -> Mux1/2
  Trigonometric Function2/1 -> Mux1/1
  Constant2/1 -> Mux1/3
  Sum/1 -> Trigonometric Function3/1, Trigonometric Function2/1
  Trigonometric Function4/1 -> Mux2/2
  Trigonometric Function1/1 -> Mux2/1
  Constant1/1 -> Mux2/3
  Trigonometric Function6/1 -> Mux3/2
  Trigonometric Function5/1 -> Mux3/1
  Constant5/1 -> Mux3/3
  Sum1/1 -> Trigonometric Function6/1, Trigonometric Function5/1
  Mux1/1 -> Matrix Concatenate/2
  Mux2/1 -> Matrix Concatenate/1
  Mux3/1 -> Matrix Concatenate/3

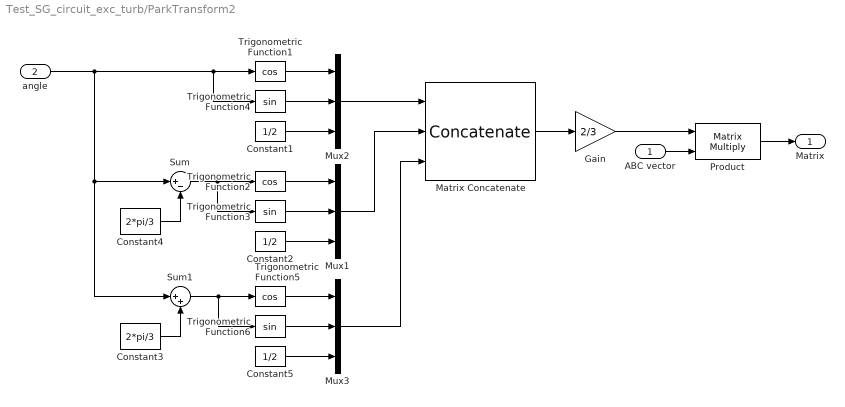
== system Test_SG_circuit_exc_turb/ParkTransform2 ==
  ABC vector : Inport
  angle : Inport  Port=2
  Constant1 : Constant  Value=1/2
  Constant2 : Constant  Value=1/2
  Constant3 : Constant  Value=2*pi/3
  Constant4 : Constant  Value=2*pi/3
  Constant5 : Constant  Value=1/2
  Gain : Gain  Gain=2/3
  Matrix Concatenate : Concatenate  NumInputs=3  Mode=Multidimensional array  ConcatenateDimension=2
  Mux1 : Mux  Inputs=3
  Mux2 : Mux  Inputs=3
  Mux3 : Mux  Inputs=3
  Product : Product  Multiplication=Matrix(*)  RndMeth=Zero
  Sum : Sum  Inputs=|+-
  Sum1 : Sum  Inputs=|++
  Trigonometric Function1 : Trigonometry  Operator=cos
  Trigonometric Function2 : Trigonometry  Operator=cos
  Trigonometric Function3 : Trigonometry
  Trigonometric Function4 : Trigonometry
  Trigonometric Function5 : Trigonometry  Operator=cos
  Trigonometric Function6 : Trigonometry
  Matrix : Outport
  wires:
  Mux3/1 -> Matrix Concatenate/3
  Mux2/1 -> Matrix Concatenate/1
  Mux1/1 -> Matrix Concatenate/2
  Sum1/1 -> Trigonometric Function5/1, Trigonometric Function6/1
  Constant5/1 -> Mux3/3
  Trigonometric Function5/1 -> Mux3/1
  Trigonometric Function6/1 -> Mux3/2
  Constant1/1 -> Mux2/3
  Trigonometric Function1/1 -> Mux2/1
  Trigonometric Function4/1 -> Mux2/2
  Sum/1 -> Trigonometric Function2/1, Trigonometric Function3/1
  Constant2/1 -> Mux1/3
  Trigonometric Function2/1 -> Mux1/1
  Trigonometric Function3/1 -> Mux1/2
  angle/1 -> Sum/1, Sum1/1, Trigonometric Function1/1, Trigonometric Function4/1
  Constant3/1 -> Sum1/2
  Constant4/1 -> Sum/2
  Gain/1 -> Product/1
  Product/1 -> Matrix/1
  ABC vector/1 -> Product/2
  Matrix Concatenate/1 -> Gain/1

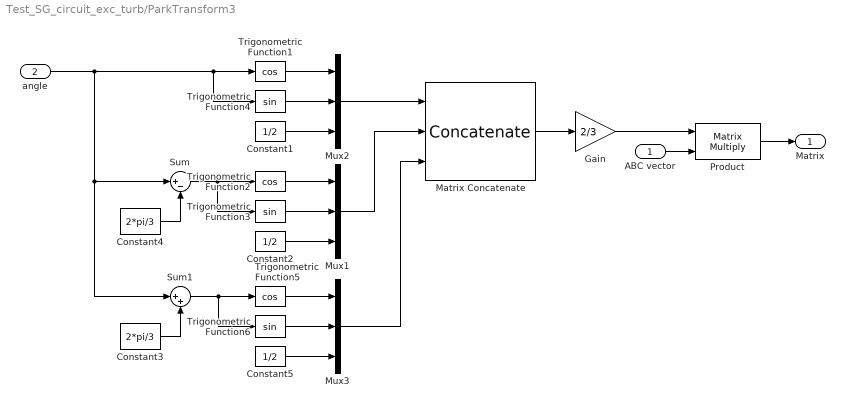
== system Test_SG_circuit_exc_turb/ParkTransform3 ==
  ABC vector : Inport
  angle : Inport  Port=2
  Constant1 : Constant  Value=1/2
  Constant2 : Constant  Value=1/2
  Constant3 : Constant  Value=2*pi/3
  Constant4 : Constant  Value=2*pi/3
  Constant5 : Constant  Value=1/2
  Gain : Gain  Gain=2/3
  Matrix Concatenate : Concatenate  NumInputs=3  Mode=Multidimensional array  ConcatenateDimension=2
  Mux1 : Mux  Inputs=3
  Mux2 : Mux  Inputs=3
  Mux3 : Mux  Inputs=3
  Product : Product  Multiplication=Matrix(*)  RndMeth=Zero
  Sum : Sum  Inputs=|+-
  Sum1 : Sum  Inputs=|++
  Trigonometric Function1 : Trigonometry  Operator=cos
  Trigonometric Function2 : Trigonometry  Operator=cos
  Trigonometric Function3 : Trigonometry
  Trigonometric Function4 : Trigonometry
  Trigonometric Function5 : Trigonometry  Operator=cos
  Trigonometric Function6 : Trigonometry
  Matrix : Outport
  wires:
  Mux3/1 -> Matrix Concatenate/3
  Mux2/1 -> Matrix Concatenate/1
  Mux1/1 -> Matrix Concatenate/2
  Sum1/1 -> Trigonometric Function5/1, Trigonometric Function6/1
  Constant5/1 -> Mux3/3
  Trigonometric Function5/1 -> Mux3/1
  Trigonometric Function6/1 -> Mux3/2
  Constant1/1 -> Mux2/3
  Trigonometric Function1/1 -> Mux2/1
  Trigonometric Function4/1 -> Mux2/2
  Sum/1 -> Trigonometric Function2/1, Trigonometric Function3/1
  Constant2/1 -> Mux1/3
  Trigonometric Function2/1 -> Mux1/1
  Trigonometric Function3/1 -> Mux1/2
  angle/1 -> Sum/1, Sum1/1, Trigonometric Function1/1, Trigonometric Function4/1
  Constant3/1 -> Sum1/2
  Constant4/1 -> Sum/2
  Gain/1 -> Product/1
  Product/1 -> Matrix/1
  ABC vector/1 -> Product/2
  Matrix Concatenate/1 -> Gain/1

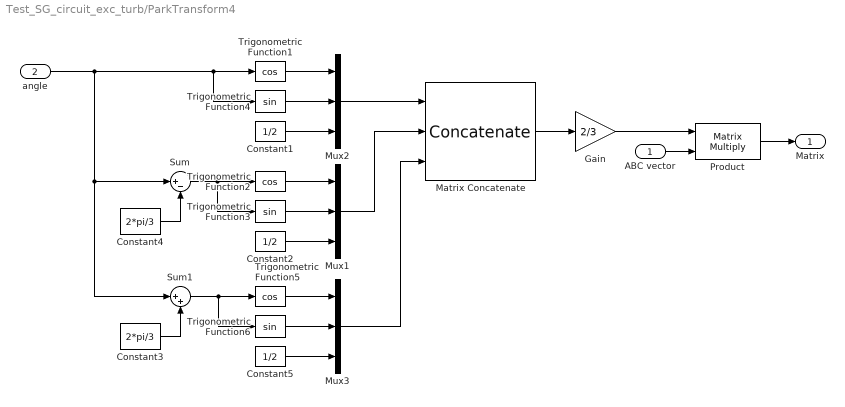
== system Test_SG_circuit_exc_turb/ParkTransform4 ==
  ABC vector : Inport
  angle : Inport  Port=2
  Constant1 : Constant  Value=1/2
  Constant2 : Constant  Value=1/2
  Constant3 : Constant  Value=2*pi/3
  Constant4 : Constant  Value=2*pi/3
  Constant5 : Constant  Value=1/2
  Gain : Gain  Gain=2/3
  Matrix Concatenate : Concatenate  NumInputs=3  Mode=Multidimensional array  ConcatenateDimension=2
  Mux1 : Mux  Inputs=3
  Mux2 : Mux  Inputs=3
  Mux3 : Mux  Inputs=3
  Product : Product  Multiplication=Matrix(*)  RndMeth=Zero
  Sum : Sum  Inputs=|+-
  Sum1 : Sum  Inputs=|++
  Trigonometric Function1 : Trigonometry  Operator=cos
  Trigonometric Function2 : Trigonometry  Operator=cos
  Trigonometric Function3 : Trigonometry
  Trigonometric Function4 : Trigonometry
  Trigonometric Function5 : Trigonometry  Operator=cos
  Trigonometric Function6 : Trigonometry
  Matrix : Outport
  wires:
  Matrix Concatenate/1 -> Gain/1
  ABC vector/1 -> Product/2
  Product/1 -> Matrix/1
  Gain/1 -> Product/1
  Constant4/1 -> Sum/2
  Constant3/1 -> Sum1/2
  angle/1 -> Trigonometric Function4/1, Trigonometric Function1/1, Sum1/1, Sum/1
  Trigonometric Function3/1 -> Mux1/2
  Trigonometric Function2/1 -> Mux1/1
  Constant2/1 -> Mux1/3
  Sum/1 -> Trigonometric Function3/1, Trigonometric Function2/1
  Trigonometric Function4/1 -> Mux2/2
  Trigonometric Function1/1 -> Mux2/1
  Constant1/1 -> Mux2/3
  Trigonometric Function6/1 -> Mux3/2
  Trigonometric Function5/1 -> Mux3/1
  Constant5/1 -> Mux3/3
  Sum1/1 -> Trigonometric Function6/1, Trigonometric Function5/1
  Mux1/1 -> Matrix Concatenate/2
  Mux2/1 -> Matrix Concatenate/1
  Mux3/1 -> Matrix Concatenate/3

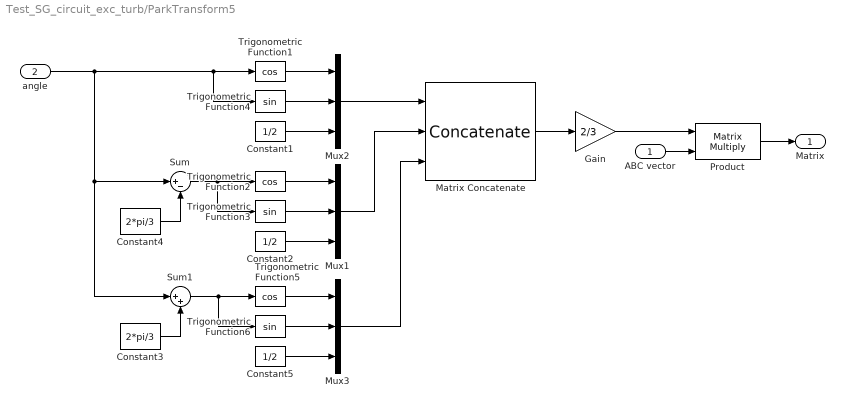
== system Test_SG_circuit_exc_turb/ParkTransform5 ==
  ABC vector : Inport
  angle : Inport  Port=2
  Constant1 : Constant  Value=1/2
  Constant2 : Constant  Value=1/2
  Constant3 : Constant  Value=2*pi/3
  Constant4 : Constant  Value=2*pi/3
  Constant5 : Constant  Value=1/2
  Gain : Gain  Gain=2/3
  Matrix Concatenate : Concatenate  NumInputs=3  Mode=Multidimensional array  ConcatenateDimension=2
  Mux1 : Mux  Inputs=3
  Mux2 : Mux  Inputs=3
  Mux3 : Mux  Inputs=3
  Product : Product  Multiplication=Matrix(*)  RndMeth=Zero
  Sum : Sum  Inputs=|+-
  Sum1 : Sum  Inputs=|++
  Trigonometric Function1 : Trigonometry  Operator=cos
  Trigonometric Function2 : Trigonometry  Operator=cos
  Trigonometric Function3 : Trigonometry
  Trigonometric Function4 : Trigonometry
  Trigonometric Function5 : Trigonometry  Operator=cos
  Trigonometric Function6 : Trigonometry
  Matrix : Outport
  wires:
  Matrix Concatenate/1 -> Gain/1
  ABC vector/1 -> Product/2
  Product/1 -> Matrix/1
  Gain/1 -> Product/1
  Constant4/1 -> Sum/2
  Constant3/1 -> Sum1/2
  angle/1 -> Trigonometric Function4/1, Trigonometric Function1/1, Sum1/1, Sum/1
  Trigonometric Function3/1 -> Mux1/2
  Trigonometric Function2/1 -> Mux1/1
  Constant2/1 -> Mux1/3
  Sum/1 -> Trigonometric Function3/1, Trigonometric Function2/1
  Trigonometric Function4/1 -> Mux2/2
  Trigonometric Function1/1 -> Mux2/1
  Constant1/1 -> Mux2/3
  Trigonometric Function6/1 -> Mux3/2
  Trigonometric Function5/1 -> Mux3/1
  Constant5/1 -> Mux3/3
  Sum1/1 -> Trigonometric Function6/1, Trigonometric Function5/1
  Mux1/1 -> Matrix Concatenate/2
  Mux2/1 -> Matrix Concatenate/1
  Mux3/1 -> Matrix Concatenate/3

== system Test_SG_circuit_exc_turb/Speed Governor ==
  note: mechanical power
  RefL : Inport
  dw : Inport  Port=2
  Gain1 : Gain  Gain=Dt
  Gain2 : Gain  Gain=1/R
  Saturation : Saturate  UpperLimit=Vmax  LowerLimit=Vmin
  Saturation1 : Saturate  UpperLimit=1
  Sum : Sum  Inputs=|+-
  Sum1 : Sum  Inputs=|+-
  Transfer Fcn (with initial outputs)1 : simulink_extras/Additional Linear/Transfer Fcn (with initial outputs)  N=[T2 1]  D=[T3 1]  Y0=P0  U0=P0
  Transfer Fcn (with initial outputs)2 : simulink_extras/Additional Linear/Transfer Fcn (with initial outputs)  N=[1]  D=[T1 1]  Y0=P0  U0=P0
  Pm : Outport
  wires:
  Gain2/1 -> Sum/2
  dw/1 -> Gain2/1, Gain1/1
  Gain1/1 -> Sum1/2
  Transfer Fcn (with initial outputs)1/1 -> Sum1/1
  Sum1/1 -> Saturation1/1
  Saturation/1 -> Transfer Fcn (with initial outputs)1/1
  Transfer Fcn (with initial outputs)2/1 -> Saturation/1
  Sum/1 -> Transfer Fcn (with initial outputs)2/1
  RefL/1 -> Sum/1
  Saturation1/1 -> Pm/1

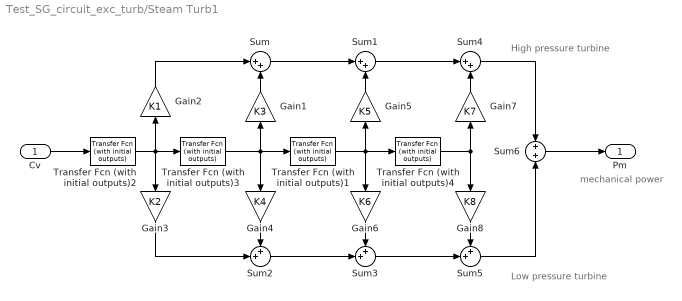
== system Test_SG_circuit_exc_turb/Steam Turb1 ==
  note: mechanical power
  note: High pressure turbine
  note: Low pressure turbine
  Cv : Inport
  Gain1 : Gain  Gain=K3
  Gain2 : Gain  Gain=K1
  Gain3 : Gain  Gain=K2
  Gain4 : Gain  Gain=K4
  Gain5 : Gain  Gain=K5
  Gain6 : Gain  Gain=K6
  Gain7 : Gain  Gain=K7
  Gain8 : Gain  Gain=K8
  Sum : Sum  Inputs=|++
  Sum1 : Sum  Inputs=|++
  Sum2 : Sum  Inputs=++|
  Sum3 : Sum  Inputs=++|
  Sum4 : Sum  Inputs=|++
  Sum5 : Sum  Inputs=++|
  Sum6 : Sum  Inputs=+|+
  Transfer Fcn (with initial outputs)1 : simulink_extras/Additional Linear/Transfer Fcn (with initial outputs)  N=[1]  D=[T6 1]  Y0=P0  U0=P0
  Transfer Fcn (with initial outputs)2 : simulink_extras/Additional Linear/Transfer Fcn (with initial outputs)  N=[1]  D=[T4 1]  Y0=P0  U0=P0
  Transfer Fcn (with initial outputs)3 : simulink_extras/Additional Linear/Transfer Fcn (with initial outputs)  N=[1]  D=[T5 1]  Y0=P0  U0=P0
  Transfer Fcn (with initial outputs)4 : simulink_extras/Additional Linear/Transfer Fcn (with initial outputs)  N=[1]  D=[T7 1]  Y0=P0  U0=P0
  Pm : Outport
  wires:
  Cv/1 -> Transfer Fcn (with initial outputs)2/1
  Transfer Fcn (with initial outputs)2/1 -> Gain2/1, Transfer Fcn (with initial outputs)3/1, Gain3/1
  Gain2/1 -> Sum/1
  Gain3/1 -> Sum2/2
  Transfer Fcn (with initial outputs)3/1 -> Gain4/1, Transfer Fcn (with initial outputs)1/1, Gain1/1
  Gain1/1 -> Sum/2
  Gain4/1 -> Sum2/1
  Gain6/1 -> Sum3/1
  Gain5/1 -> Sum1/2
  Transfer Fcn (with initial outputs)1/1 -> Gain5/1, Transfer Fcn (with initial outputs)4/1, Gain6/1
  Sum2/1 -> Sum3/2
  Sum/1 -> Sum1/1
  Sum1/1 -> Sum4/1
  Sum3/1 -> Sum5/2
  Transfer Fcn (with initial outputs)4/1 -> Gain8/1, Gain7/1
  Gain7/1 -> Sum4/2
  Gain8/1 -> Sum5/1
  Sum4/1 -> Sum6/1
  Sum5/1 -> Sum6/2
  Sum6/1 -> Pm/1

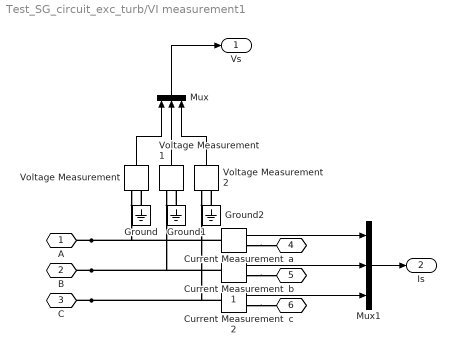
== system Test_SG_circuit_exc_turb/VI measurement1 ==
  Current Measurement : powerlib/Measurements/Current Measurement  PhasorSimulation=off  OutputType=Complex  PSBequivalent=0
  Current Measurement1 : powerlib/Measurements/Current Measurement  PhasorSimulation=off  OutputType=Complex  PSBequivalent=0
  Current Measurement2 : powerlib/Measurements/Current Measurement  PhasorSimulation=off  OutputType=Complex  PSBequivalent=0
  Ground : powerlib/Elements/Ground  LConnTagsString=a
  Ground1 : powerlib/Elements/Ground  LConnTagsString=a
  Ground2 : powerlib/Elements/Ground  LConnTagsString=a
  Mux : Mux  Inputs=3
  Mux1 : Mux  Inputs=3
  Voltage Measurement : powerlib/Measurements/Voltage Measurement  PhasorSimulation=off  OutputType=Complex  PSBequivalent=0
  Voltage Measurement1 : powerlib/Measurements/Voltage Measurement  PhasorSimulation=off  OutputType=Complex  PSBequivalent=0
  Voltage Measurement2 : powerlib/Measurements/Voltage Measurement  PhasorSimulation=off  OutputType=Complex  PSBequivalent=0
  A : PMIOPort  Side=Left
  B : PMIOPort  Port=2  Side=Left
  C : PMIOPort  Port=3  Side=Left
  a : PMIOPort  Port=4  Side=Right
  b : PMIOPort  Port=5  Side=Right
  c : PMIOPort  Port=6  Side=Right
  Vs : Outport
  Is : Outport  Port=2
  wires:
  Current Measurement1/1 -> Mux1/2
  Current Measurement/1 -> Mux1/1
  Voltage Measurement/1 -> Mux/1
  Current Measurement2/1 -> Mux1/3
  Voltage Measurement2/1 -> Mux/3
  Voltage Measurement1/1 -> Mux/2
  Mux/1 -> Vs/1
  Mux1/1 -> Is/1
  connections:
  Ground2/LConn1 -- Voltage Measurement2/LConn2
  Ground1/LConn1 -- Voltage Measurement1/LConn2
  Current Measurement2/RConn1 -- c/RConn1
  Ground/LConn1 -- Voltage Measurement/LConn2
  Current Measurement/RConn1 -- a/RConn1
  Current Measurement1/RConn1 -- b/RConn1
  B/RConn1 -- Voltage Measurement1/LConn1 -- Current Measurement1/LConn1
  C/RConn1 -- Voltage Measurement2/LConn1 -- Current Measurement2/LConn1
  A/RConn1 -- Current Measurement/LConn1 -- Voltage Measurement/LConn1

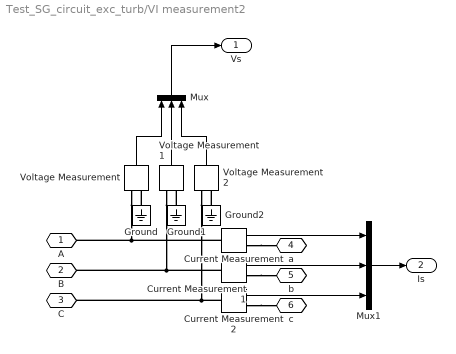
== system Test_SG_circuit_exc_turb/VI measurement2 ==
  Current Measurement : powerlib/Measurements/Current Measurement  PhasorSimulation=off  OutputType=Complex  PSBequivalent=0
  Current Measurement1 : powerlib/Measurements/Current Measurement  PhasorSimulation=off  OutputType=Complex  PSBequivalent=0
  Current Measurement2 : powerlib/Measurements/Current Measurement  PhasorSimulation=off  OutputType=Complex  PSBequivalent=0
  Ground : powerlib/Elements/Ground  LConnTagsString=a
  Ground1 : powerlib/Elements/Ground  LConnTagsString=a
  Ground2 : powerlib/Elements/Ground  LConnTagsString=a
  Mux : Mux  Inputs=3
  Mux1 : Mux  Inputs=3
  Voltage Measurement : powerlib/Measurements/Voltage Measurement  PhasorSimulation=off  OutputType=Complex  PSBequivalent=0
  Voltage Measurement1 : powerlib/Measurements/Voltage Measurement  PhasorSimulation=off  OutputType=Complex  PSBequivalent=0
  Voltage Measurement2 : powerlib/Measurements/Voltage Measurement  PhasorSimulation=off  OutputType=Complex  PSBequivalent=0
  A : PMIOPort  Side=Left
  B : PMIOPort  Port=2  Side=Left
  C : PMIOPort  Port=3  Side=Left
  a : PMIOPort  Port=4  Side=Right
  b : PMIOPort  Port=5  Side=Right
  c : PMIOPort  Port=6  Side=Right
  Vs : Outport
  Is : Outport  Port=2
  wires:
  Mux1/1 -> Is/1
  Mux/1 -> Vs/1
  Voltage Measurement1/1 -> Mux/2
  Voltage Measurement2/1 -> Mux/3
  Current Measurement2/1 -> Mux1/3
  Voltage Measurement/1 -> Mux/1
  Current Measurement/1 -> Mux1/1
  Current Measurement1/1 -> Mux1/2
  connections:
  Voltage Measurement/LConn1 -- Current Measurement/LConn1 -- A/RConn1
  Current Measurement2/LConn1 -- Voltage Measurement2/LConn1 -- C/RConn1
  Current Measurement1/LConn1 -- Voltage Measurement1/LConn1 -- B/RConn1
  Current Measurement1/RConn1 -- b/RConn1
  Current Measurement/RConn1 -- a/RConn1
  Ground/LConn1 -- Voltage Measurement/LConn2
  Current Measurement2/RConn1 -- c/RConn1
  Ground1/LConn1 -- Voltage Measurement1/LConn2
  Ground2/LConn1 -- Voltage Measurement2/LConn2

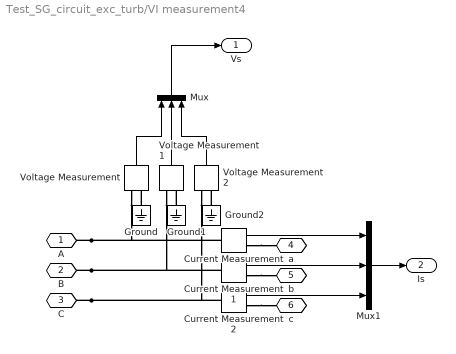
== system Test_SG_circuit_exc_turb/VI measurement4 ==
  Current Measurement : powerlib/Measurements/Current Measurement  PhasorSimulation=off  OutputType=Complex  PSBequivalent=0
  Current Measurement1 : powerlib/Measurements/Current Measurement  PhasorSimulation=off  OutputType=Complex  PSBequivalent=0
  Current Measurement2 : powerlib/Measurements/Current Measurement  PhasorSimulation=off  OutputType=Complex  PSBequivalent=0
  Ground : powerlib/Elements/Ground  LConnTagsString=a
  Ground1 : powerlib/Elements/Ground  LConnTagsString=a
  Ground2 : powerlib/Elements/Ground  LConnTagsString=a
  Mux : Mux  Inputs=3
  Mux1 : Mux  Inputs=3
  Voltage Measurement : powerlib/Measurements/Voltage Measurement  PhasorSimulation=off  OutputType=Complex  PSBequivalent=0
  Voltage Measurement1 : powerlib/Measurements/Voltage Measurement  PhasorSimulation=off  OutputType=Complex  PSBequivalent=0
  Voltage Measurement2 : powerlib/Measurements/Voltage Measurement  PhasorSimulation=off  OutputType=Complex  PSBequivalent=0
  A : PMIOPort  Side=Left
  B : PMIOPort  Port=2  Side=Left
  C : PMIOPort  Port=3  Side=Left
  a : PMIOPort  Port=4  Side=Right
  b : PMIOPort  Port=5  Side=Right
  c : PMIOPort  Port=6  Side=Right
  Vs : Outport
  Is : Outport  Port=2
  wires:
  Current Measurement1/1 -> Mux1/2
  Current Measurement/1 -> Mux1/1
  Voltage Measurement/1 -> Mux/1
  Current Measurement2/1 -> Mux1/3
  Voltage Measurement2/1 -> Mux/3
  Voltage Measurement1/1 -> Mux/2
  Mux/1 -> Vs/1
  Mux1/1 -> Is/1
  connections:
  Ground2/LConn1 -- Voltage Measurement2/LConn2
  Ground1/LConn1 -- Voltage Measurement1/LConn2
  Current Measurement2/RConn1 -- c/RConn1
  Ground/LConn1 -- Voltage Measurement/LConn2
  Current Measurement/RConn1 -- a/RConn1
  Current Measurement1/RConn1 -- b/RConn1
  B/RConn1 -- Voltage Measurement1/LConn1 -- Current Measurement1/LConn1
  C/RConn1 -- Voltage Measurement2/LConn1 -- Current Measurement2/LConn1
  A/RConn1 -- Current Measurement/LConn1 -- Voltage Measurement/LConn1

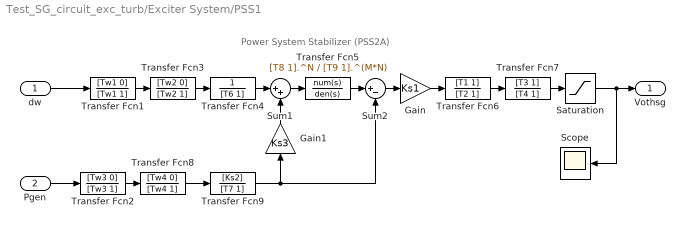
== system Test_SG_circuit_exc_turb/Exciter System/PSS1 ==
  note: Power System Stabilizer (PSS2A)
  dw : Inport
  Pgen : Inport  Port=2
  Gain : Gain  Gain=Ks1
  Gain1 : Gain  Gain=Ks3
  Saturation : Saturate  UpperLimit=Vstmax  LowerLimit=Vstmin
  Scope : Scope
  Sum1 : Sum  Inputs=|++
  Sum2 : Sum  Inputs=|+-
  Transfer Fcn1 : TransferFcn  Numerator=[Tw1 0]  Denominator=[Tw1 1]
  Transfer Fcn2 : TransferFcn  Numerator=[Tw3 0]  Denominator=[Tw3 1]
  Transfer Fcn3 : TransferFcn  Numerator=[Tw2 0]  Denominator=[Tw2 1]
  Transfer Fcn4 : TransferFcn  Denominator=[T6 1]
  Transfer Fcn5 : TransferFcn  Numerator=[T8 1].^N  Denominator=[T9 1].^(M*N)
  Transfer Fcn6 : TransferFcn  Numerator=[T1 1]  Denominator=[T2 1]
  Transfer Fcn7 : TransferFcn  Numerator=[T3 1]  Denominator=[T4 1]
  Transfer Fcn8 : TransferFcn  Numerator=[Tw4 0]  Denominator=[Tw4 1]
  Transfer Fcn9 : TransferFcn  Numerator=[Ks2]  Denominator=[T7 1]
  Vothsg : Outport
  wires:
  Transfer Fcn9/1 -> Sum2/2, Gain1/1
  Gain1/1 -> Sum1/2
  Transfer Fcn8/1 -> Transfer Fcn9/1
  Transfer Fcn2/1 -> Transfer Fcn8/1
  Pgen/1 -> Transfer Fcn2/1
  Saturation/1 -> Scope/1, Vothsg/1
  Transfer Fcn7/1 -> Saturation/1
  Transfer Fcn6/1 -> Transfer Fcn7/1
  Gain/1 -> Transfer Fcn6/1
  Sum2/1 -> Gain/1
  Transfer Fcn5/1 -> Sum2/1
  Sum1/1 -> Transfer Fcn5/1
  Transfer Fcn4/1 -> Sum1/1
  Transfer Fcn3/1 -> Transfer Fcn4/1
  Transfer Fcn1/1 -> Transfer Fcn3/1
  dw/1 -> Transfer Fcn1/1

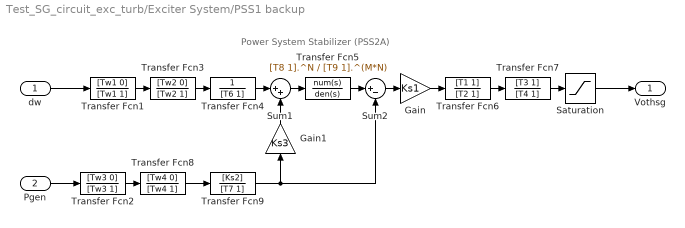
== system Test_SG_circuit_exc_turb/Exciter System/PSS1 backup ==
  note: Power System Stabilizer (PSS2A)
  dw : Inport
  Pgen : Inport  Port=2
  Gain : Gain  Gain=Ks1
  Gain1 : Gain  Gain=Ks3
  Saturation : Saturate  UpperLimit=Vstmax  LowerLimit=Vstmin
  Sum1 : Sum  Inputs=|++
  Sum2 : Sum  Inputs=|+-
  Transfer Fcn1 : TransferFcn  Numerator=[Tw1 0]  Denominator=[Tw1 1]
  Transfer Fcn2 : TransferFcn  Numerator=[Tw3 0]  Denominator=[Tw3 1]
  Transfer Fcn3 : TransferFcn  Numerator=[Tw2 0]  Denominator=[Tw2 1]
  Transfer Fcn4 : TransferFcn  Denominator=[T6 1]
  Transfer Fcn5 : TransferFcn  Numerator=[T8 1].^N  Denominator=[T9 1].^(M*N)
  Transfer Fcn6 : TransferFcn  Numerator=[T1 1]  Denominator=[T2 1]
  Transfer Fcn7 : TransferFcn  Numerator=[T3 1]  Denominator=[T4 1]
  Transfer Fcn8 : TransferFcn  Numerator=[Tw4 0]  Denominator=[Tw4 1]
  Transfer Fcn9 : TransferFcn  Numerator=[Ks2]  Denominator=[T7 1]
  Vothsg : Outport
  wires:
  dw/1 -> Transfer Fcn1/1
  Transfer Fcn1/1 -> Transfer Fcn3/1
  Transfer Fcn3/1 -> Transfer Fcn4/1
  Transfer Fcn4/1 -> Sum1/1
  Sum1/1 -> Transfer Fcn5/1
  Transfer Fcn5/1 -> Sum2/1
  Sum2/1 -> Gain/1
  Gain/1 -> Transfer Fcn6/1
  Transfer Fcn6/1 -> Transfer Fcn7/1
  Transfer Fcn7/1 -> Saturation/1
  Saturation/1 -> Vothsg/1
  Pgen/1 -> Transfer Fcn2/1
  Transfer Fcn2/1 -> Transfer Fcn8/1
  Transfer Fcn8/1 -> Transfer Fcn9/1
  Gain1/1 -> Sum1/2
  Transfer Fcn9/1 -> Gain1/1, Sum2/2
